simulink model "ZumoTrackSandip"  (R2014b)
settings: Solver=ode45  StartTime=0.0  StopTime=inf  RelTol=1e-3
InitFcn:
  | z = comms.Bt(RobotID.ZUMO_ADAFRUIT_32B0);
  | z.reset();
  | z.init();
  | %z.write(320*((255-1)/(640-1)),1);
  | %z.write(240*((255-1)/(480-1)),1);
  | 
  | clear detectMinions2
undefined symbols (not defined in the file or in its folder): IsPositionTracked, IsSkeletonTracked, JointDepthIndices, JointImageIndices, JointTrackingState, JointWorldCoordinates, none, PositionDepthIndices, PositionImageIndices, PositionWorldCoordinates, SegmentationData, SkeletonTrackingID, videoinput
libraries: visiontextngfix x2, imaqlib x1, simulink x1, hostCommsLib x1, visionsinks x1
settings Model: Creator=gsalhotr  LastModifiedBy=sandip

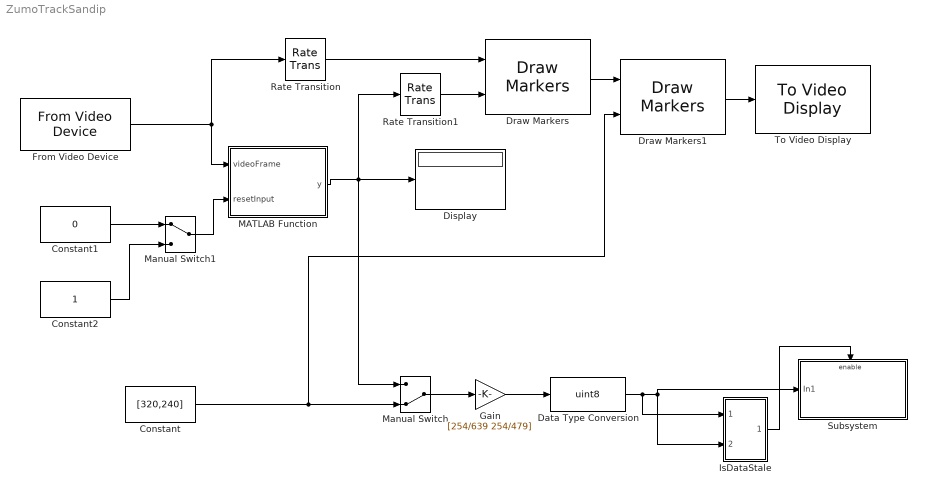
== system ZumoTrackSandip ==
  Constant : Constant  Value=[320,240]  OutDataTypeStr=single  SampleTime=0.01
  Constant1 : Constant  Value=0  OutDataTypeStr=single  SampleTime=0.01
  Constant2 : Constant  OutDataTypeStr=single  SampleTime=0.01
  Data Type Conversion : DataTypeConversion  OutDataTypeStr=uint8
  Display : Display
  Draw Markers : visiontextngfix/Draw Markers  shape=Circle  size=5  fill=on  fillClrSource=Specify via dialog  display=User-specified value  intensity=200  color=[255 0 0]  opacity=0.6  viewport=Entire image  antialiasing=off  inType=Obsolete  imagePorts=One multidimensional signal  prodOutputMode=Binary point scaling  prodOutputWordLength=32  prodOutputFracLength=14  memoryMode=Specify word length  memoryWordLength=16  memoryFracLength=14  roundingMode=Floor  overflowMode=off
  Draw Markers1 : visiontextngfix/Draw Markers  shape=X-mark  size=5  fill=on  fillClrSource=Specify via dialog  display=User-specified value  intensity=200  color=[255 0 0]  opacity=0.6  viewport=Entire image  antialiasing=off  inType=Obsolete  imagePorts=One multidimensional signal  prodOutputMode=Binary point scaling  prodOutputWordLength=32  prodOutputFracLength=14  memoryMode=Specify word length  memoryWordLength=16  memoryFracLength=14  roundingMode=Floor  overflowMode=off
  From Video Device : imaqlib/From Video Device  DeviceMenu=winvideo 1 (USB2.0 HD UVC WebCam)  Device=winvideo 2 (Logitech QuickCam Pro 9000)  ObjConstructor=videoinput('winvideo', 2)  VideoFormatMenu=MJPG_1280x720  VideoFormat=I420_640x480  VideoSource=input1  ROIPosition=[0 0 480 640]  EnableHWTrigger=off  TriggerConfiguration=none/none  SampleTime=1/30  OutputPortsMode=One multidimensional signal  DataType=single  CanDoHWTrigger=no  ReturnedColorSpace=rgb  BlockHandle=1921.0006  ROIWidth=640  ROIHeight=480  ROIColumn=0  ROIRow=0  EngXMLPath=C:\Program Files\MATLAB\R2014b\toolbox\imaq\imaq\private  DevXMLPath=C:\MATLAB\SupportPackages\R2014b\osgenericvideointerface\toolbox\imaq\supportpackages\genericvideo\adaptor\win64  EngLibPath=C:\Program Files\MATLAB\R2014b\toolbox\imaq\imaqblks\imaqmex\win64  ColorSpace=rgb  BayerSensorAlignment=grbg  AllMetadata=IsPositionTracked;IsSkeletonTracked;JointDepthIndices;JointImageIndices;JointTrackingState;JointWorldCoordinates;PositionDepthIndices;PositionImageIndices;PositionWorldCoordinates;SegmentationData;SkeletonTrackingID
  Gain : Gain  Gain=[254/639 254/479]
  IsDataStale : Subsystem
  MATLAB Function : MATLAB Function  TreatAsAtomicUnit=on
  Manual Switch : ManualSwitch  CurrentSetting=0
  Manual Switch1 : ManualSwitch
  Rate Transition : RateTransition  OutPortSampleTime=0.1
  Rate Transition1 : RateTransition  OutPortSampleTime=0.1
  Subsystem : Subsystem
  To Video Display : visionsinks/To Video Display  inputType=Obsolete  imagePorts=One multidimensional signal  OutputDevice=On-screen video monitor  fullScreen=off  videoWindowX=1186  videoWindowY=358  saveWindowSize=off  videoWindowWidth=640  videoWindowHeight=480  dataOrg=Column-major  openAtMdlStart=on  isWindowOpen=off  inputColorFormat=RGB
  wires:
  From Video Device/1 -> Rate Transition/1, MATLAB Function/1(videoFrame)
  Rate Transition/1 -> Draw Markers/1
  Rate Transition1/1 -> Draw Markers/2
  MATLAB Function/1(y) -> Manual Switch/1, Display/1, Rate Transition1/1
  Manual Switch/1 -> Gain/1
  Data Type Conversion/1 -> IsDataStale/1(In1), IsDataStale/2(In2), Subsystem/1(In1)
  IsDataStale/1(Out1) -> Subsystem/Enable
  Constant/1 -> Draw Markers1/2, Manual Switch/2
  Gain/1 -> Data Type Conversion/1
  Draw Markers/1 -> Draw Markers1/1
  Draw Markers1/1 -> To Video Display/1
  Manual Switch1/1 -> MATLAB Function/2(resetInput)
  Constant1/1 -> Manual Switch1/1
  Constant2/1 -> Manual Switch1/2

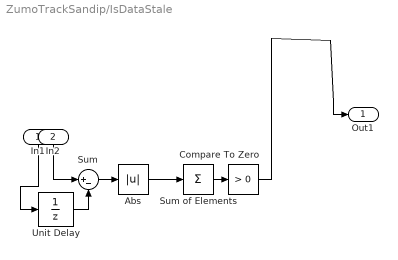
== system ZumoTrackSandip/IsDataStale ==
  In1 : Inport
  In2 : Inport  Port=2
  Abs : Abs
  Compare To Zero : simulink/Logic and Bit Operations/Compare To Zero  relop=>  OutDataTypeStr=boolean
  Sum : Sum  Inputs=|+-
  Sum of Elements : Sum  Inputs=+
  Unit Delay : UnitDelay  SampleTime=-1
  Out1 : Outport
  wires:
  In2/1 -> Sum/1
  In1/1 -> Unit Delay/1
  Compare To Zero/1 -> Out1/1
  Abs/1 -> Sum of Elements/1
  Sum/1 -> Abs/1
  Unit Delay/1 -> Sum/2
  Sum of Elements/1 -> Compare To Zero/1

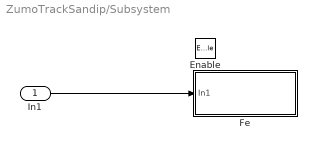
== system ZumoTrackSandip/Subsystem ==
  In1 : Inport
  Enable : EnablePort
  Fe : Subsystem  TreatAsAtomicUnit=on
  wires:
  In1/1 -> Fe/1(In1)

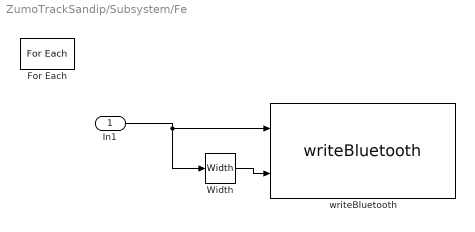
== system ZumoTrackSandip/Subsystem/Fe ==
  In1 : Inport  Partition=on  PartitionDimension=2  PartitionWidth=1
  For Each : ForEach  DisableCoverage=on  IndexMode=One-based
  Width : Width
  writeBluetooth : hostCommsLib/writeBluetooth  robotId=RobotID.ZUMO_ADAFRUIT_32B0
  wires:
  In1/1 -> Width/1, writeBluetooth/1
  Width/1 -> writeBluetooth/2

== matlab function ZumoTrackSandip/MATLAB Function ==
  data: videoFrame input; y output; resetInput input
function y = fcn(videoFrame, resetInput)
%#codegen
persistent initFlag;
if isempty(initFlag) || resetInput
    initFlag = 1;
end
y = ones([1 2], 'single');
coder.extrinsic('detectMinions2');
coder.extrinsic('vision.PointTracker');

y = detectMinions2(videoFrame, initFlag);
initFlag = 0;

end
